simulink subsystem "railCarBrakeSubSystem"  (R2025a)
settings: Solver=VariableStepAuto  StartTime=0.0  StopTime=10.0  RelTol=1e-3
model mask{reservoir_temperature=70, reservoir_temperature_unit=degF, p_init=air_pressure, p_init_unit=psi, r_volume=10, r_volume_unit=gal, bc_volume=4, bc_volume_unit=gal, bc_pressure=14.69, bc_pressure_unit=psi, length=50, length_unit=ft, area=1.23, area_unit=in^2, Dh=1.25, Dh_unit=in}
  mask prompts: reservoir_temperature "physmod:simscape:library:comments:gas:elements:reservoir:reservoir_temperature"; p_init "physmod:simscape:library:comments:gas:elements:pipe:p_init"; r_volume "Volume"; bc_volume "Volume"; bc_pressure "Pressure"; length "Pipe length"; area "Cross-sectional area"; Dh "Hydraulic diameter"
libraries: fl_lib x17, nesl_utility x10, SimscapeFluids_lib x5
settings Model: Creator=adam  LastModifiedBy=adam
settings OptimizationCC: ReuseModelBlockBuffer=off
settings RTWCC: GPUComputeCapability=3.5

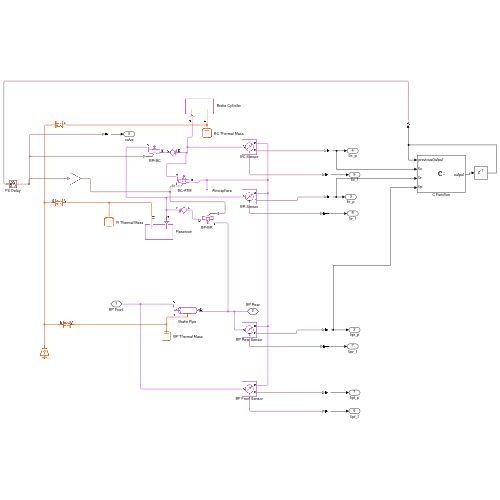
[thumbnail: Simulink's stored preview of the top-level diagram]
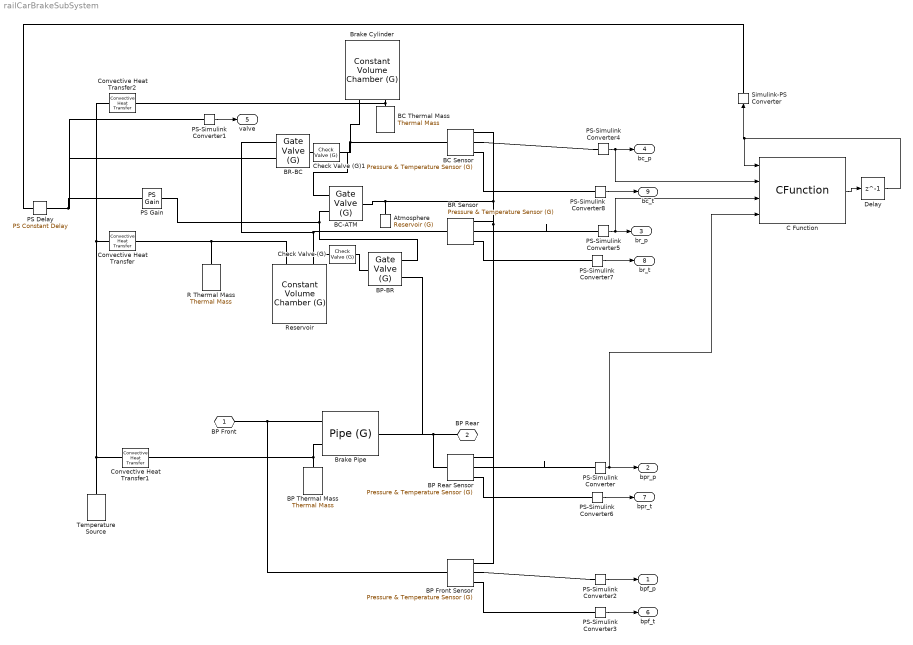
== system railCarBrakeSubSystem ==
  Atmosphere : fl_lib/Gas/Elements/Reservoir (G)  pressure_spec=foundation.enum.pressure_spec.atmospheric  reservoir_pressure=0.101325 MPa  reservoir_temperature=reservoir_temperature degF  area_A=10 ft^2
  BC Sensor : fl_lib/Gas/Sensors/Pressure & Temperature Sensor (G)  reference=foundation.enum.MeasurementReference.difference  pressure=true  pressure_spec=foundation.enum.PressureMeasementSpec.Absolute  temperature=true
      settings: InternalSimscapePortConfiguration="{\"Bottom\":[{\"id\":\"T\",\"label\":\"T\",\"type\":\"output\"}],\"Left\":[{\"id\":\"A\",\"label\":\"A\",\"type\":\"foundation.gas.gas\"}],\"Right\":[{\"id\":\"B\",\"label\":\"B\",\"type\":\"foundation.gas.gas\"},{\"id\":\"P\",\"label\":\"P\",\"type\":\"output\"}],\"Top\":[]}"
  BC Thermal Mass : fl_lib/Thermal/Thermal Elements/Thermal Mass  mass_type=foundation.enum.constant_variable.constant  mass=100 kg  sp_heat=447 J/(K*kg)  mass_min=1e-6 kg  num_ports=foundation.enum.numPorts2.one  m_specify=off  m_priority=High  m=1 kg  m_nominal_specify=off  m_nominal_value=1  m_nominal_unit=kg  T_specify=on  T_priority=High  T=reservoir_temperature degF  T_nominal_specify=off  T_nominal_value=1  T_nominal_unit=K  Q_specify=off  Q_priority=None  Q=0 W  Q_nominal_specify=off  Q_nominal_value=1  Q_nominal_unit=W
  BC-ATM : SimscapeFluids_lib/Gas/Valves & Orifices/Flow Control Valves/Gate Valve (G)  diam_orifice=1.25 in  valve_parameterization=fluids.gas.valves_orifices.flow_control_valves.enum.OrificeParameterization.Cv  Cd=0.64  Cv_max=4  xT_Cv=0.7  Kv_max=3.6  xT_Kv=0.7  C_max=12 l/(bar*s)  B_crit_linear=0.3  m=0.5  T_ref_C=293.15 K  rho_ref_C=1.185 kg/m^3  leakage_fraction=1e-7  smoothing_factor=0.0001  B_lam=0.999  area=1.23 in^2  x0=0
      settings: InternalSimscapePortConfiguration="{\"Bottom\":[],\"Left\":[{\"id\":\"A\",\"label\":\"A\",\"type\":\"foundation.gas.gas\"},{\"id\":\"L\",\"label\":\"L\",\"type\":\"input\"}],\"Right\":[{\"id\":\"B\",\"label\":\"B\",\"type\":\"foundation.gas.gas\"}],\"Top\":[]}"
  BP Front Sensor : fl_lib/Gas/Sensors/Pressure & Temperature Sensor (G)  reference=foundation.enum.MeasurementReference.difference  pressure=true  pressure_spec=foundation.enum.PressureMeasementSpec.Absolute  temperature=true
      settings: InternalSimscapePortConfiguration="{\"Bottom\":[{\"id\":\"T\",\"label\":\"T\",\"type\":\"output\"}],\"Left\":[{\"id\":\"A\",\"label\":\"A\",\"type\":\"foundation.gas.gas\"}],\"Right\":[{\"id\":\"B\",\"label\":\"B\",\"type\":\"foundation.gas.gas\"},{\"id\":\"P\",\"label\":\"P\",\"type\":\"output\"}],\"Top\":[]}"
  BP Rear Sensor : fl_lib/Gas/Sensors/Pressure & Temperature Sensor (G)  reference=foundation.enum.MeasurementReference.difference  pressure=true  pressure_spec=foundation.enum.PressureMeasementSpec.Absolute  temperature=true
      settings: InternalSimscapePortConfiguration="{\"Bottom\":[{\"id\":\"T\",\"label\":\"T\",\"type\":\"output\"}],\"Left\":[{\"id\":\"A\",\"label\":\"A\",\"type\":\"foundation.gas.gas\"}],\"Right\":[{\"id\":\"B\",\"label\":\"B\",\"type\":\"foundation.gas.gas\"},{\"id\":\"P\",\"label\":\"P\",\"type\":\"output\"}],\"Top\":[]}"
  BP Thermal Mass : fl_lib/Thermal/Thermal Elements/Thermal Mass  mass_type=foundation.enum.constant_variable.constant  mass=2.27*50 lbm  sp_heat=447 J/(K*kg)  mass_min=1e-6 kg  num_ports=foundation.enum.numPorts2.one  m_specify=off  m_priority=High  m=1 kg  m_nominal_specify=off  m_nominal_value=1  m_nominal_unit=kg  T_specify=on  T_priority=High  T=reservoir_temperature degF  T_nominal_specify=off  T_nominal_value=1  T_nominal_unit=K  Q_specify=off  Q_priority=None  Q=0 W  Q_nominal_specify=off  Q_nominal_value=1  Q_nominal_unit=W
  BP-BR : SimscapeFluids_lib/Gas/Valves & Orifices/Flow Control Valves/Gate Valve (G)  diam_orifice=1.25 in  valve_parameterization=fluids.gas.valves_orifices.flow_control_valves.enum.OrificeParameterization.Cv  Cd=0.64  Cv_max=4  xT_Cv=0.7  Kv_max=3.6  xT_Kv=0.7  C_max=12 l/(bar*s)  B_crit_linear=0.3  m=0.5  T_ref_C=293.15 K  rho_ref_C=1.185 kg/m^3  leakage_fraction=1e-7  smoothing_factor=0.0001  B_lam=0.999  area=1.23 in^2  x0=0
      settings: InternalSimscapePortConfiguration="{\"Bottom\":[],\"Left\":[{\"id\":\"A\",\"label\":\"A\",\"type\":\"foundation.gas.gas\"},{\"id\":\"L\",\"label\":\"L\",\"type\":\"input\"}],\"Right\":[{\"id\":\"B\",\"label\":\"B\",\"type\":\"foundation.gas.gas\"}],\"Top\":[]}"
  BR Sensor : fl_lib/Gas/Sensors/Pressure & Temperature Sensor (G)  reference=foundation.enum.MeasurementReference.difference  pressure=true  pressure_spec=foundation.enum.PressureMeasementSpec.Absolute  temperature=true
      settings: InternalSimscapePortConfiguration="{\"Bottom\":[{\"id\":\"T\",\"label\":\"T\",\"type\":\"output\"}],\"Left\":[{\"id\":\"A\",\"label\":\"A\",\"type\":\"foundation.gas.gas\"}],\"Right\":[{\"id\":\"B\",\"label\":\"B\",\"type\":\"foundation.gas.gas\"},{\"id\":\"P\",\"label\":\"P\",\"type\":\"output\"}],\"Top\":[]}"
  BR-BC : SimscapeFluids_lib/Gas/Valves & Orifices/Flow Control Valves/Gate Valve (G)  diam_orifice=1.25 in  valve_parameterization=fluids.gas.valves_orifices.flow_control_valves.enum.OrificeParameterization.Cv  Cd=0.64  Cv_max=4  xT_Cv=0.7  Kv_max=3.6  xT_Kv=0.7  C_max=12 l/(bar*s)  B_crit_linear=0.3  m=0.5  T_ref_C=293.15 K  rho_ref_C=1.185 kg/m^3  leakage_fraction=1e-7  smoothing_factor=0.0001  B_lam=0.999  area=1.23 in^2  x0=0
      settings: InternalSimscapePortConfiguration="{\"Bottom\":[],\"Left\":[{\"id\":\"A\",\"label\":\"A\",\"type\":\"foundation.gas.gas\"},{\"id\":\"L\",\"label\":\"L\",\"type\":\"input\"}],\"Right\":[{\"id\":\"B\",\"label\":\"B\",\"type\":\"foundation.gas.gas\"}],\"Top\":[]}"
  Brake Cylinder : fl_lib/Gas/Elements/Constant Volume Chamber (G)  volume=bc_volume gal  num_ports=foundation.enum.num_ports.one  area_A=0.11 in^2  area_B=0.11 in^2  area_C=0.01 m^2  area_D=0.01 m^2  p_I_specify=on  p_I_priority=High  p_I=bc_pressure psi  p_I_nominal_specify=off  p_I_nominal_value=1  p_I_nominal_unit=MPa  T_I_specify=on  T_I_priority=High  T_I=reservoir_temperature degF  T_I_nominal_specify=off  T_I_nominal_value=1  T_I_nominal_unit=K  rho_I_specify=off  rho_I_priority=None  rho_I=1.2 kg/m^3  rho_I_nominal_specify=off  rho_I_nominal_value=1  rho_I_nominal_unit=kg/m^3
      settings: InternalSimscapePortConfiguration="{\"Bottom\":[],\"Left\":[{\"id\":\"A\",\"label\":\"A\",\"type\":\"foundation.gas.gas\"},{\"id\":\"H\",\"label\":\"H\",\"type\":\"foundation.thermal.thermal\"}],\"Right\":[],\"Top\":[]}"
  Brake Pipe : fl_lib/Gas/Elements/Pipe (G)  length=length ft  area=area in^2  Dh=Dh in  length_add=0.1 m  roughness=15e-6 m  Re_lam=2000  Re_tur=4000  shape_factor=64  Nu_lam=3.66  dynamic_compressibility=true  inertia=false  p_init=p_init psi  p_init_priority=foundation.enum.Priority.High  T_init=reservoir_temperature degF  T_init_priority=foundation.enum.Priority.High  mdot_init=0 kg/s  mdot_init_priority=foundation.enum.Priority.High  p_nominal=0.101325 MPa  T_nominal=293.15 K
  C Function : CFunction  OutputCode=|  GenerateCodeAsIs=off  CodegenOutputCode=|  CustomCodeSettingLocation=ModelConfigurationParameters
      OutputCode=|
      | // 1 = Apply
      | // 0 = Lap
      | // -1 = Release
      | 
      | if (bp > br + 1.5) {
      |     // BP-BR and BC-ATM
      |     output = -1;
      | } else if (bp < br - 1.5) {
      |     // BR-BC
      |     output = 1;
      | } else {
      |     output = 0;   
      | }
      CodegenOutputCode=|
      | // 1 = Apply
      | // 0 = Lap
      | // -1 = Release
      | 
      | if (bp > br + 1.5) {
      |     // BP-BR and BC-ATM
      |     output = -1;
      | } else if (bp < br - 1.5) {
      |     // BR-BC
      |     output = 1;
      | } else {
      |     output = 0;   
      | }
  Check Valve (G) : SimscapeFluids_lib/Gas/Valves & Orifices/Directional Control Valves/Check Valve (G)  opening_pressure_spec=fluids.gas.valves_orifices.enum.PressureControlSpec.PressureDifference  p_crack_differential=0.1 psi  p_crack_gauge=0.1 MPa  press_max_differential=0.25 psi  press_max_gauge=0.2 MPa  valve_parameterization=fluids.gas.valves_orifices.enum.OrificeParameterization.Cv  Cv_max=4  xT_Cv=0.7  Kv_max=3.6  xT_Kv=0.7  C_max=12 l/(bar*s)  B_crit_linear=0.3  m=0.5  T_ref_C=293.15 K  rho_ref_C=1.185 kg/m^3  orifice_area_max=1e-4 m^2  Cd=0.64  leakage_fraction=1e-7  smoothing_factor=0.01  B_lam=0.999  area=1.23 in^2
      settings: InternalSimscapePortConfiguration="{\"Bottom\":[],\"Left\":[{\"id\":\"A\",\"label\":\"A\",\"type\":\"foundation.gas.gas\"}],\"Right\":[{\"id\":\"B\",\"label\":\"B\",\"type\":\"foundation.gas.gas\"}],\"Top\":[]}"
  Check Valve (G)1 : SimscapeFluids_lib/Gas/Valves & Orifices/Directional Control Valves/Check Valve (G)  opening_pressure_spec=fluids.gas.valves_orifices.enum.PressureControlSpec.PressureDifference  p_crack_differential=0.1 psi  p_crack_gauge=0.1 MPa  press_max_differential=0.25 psi  press_max_gauge=0.2 MPa  valve_parameterization=fluids.gas.valves_orifices.enum.OrificeParameterization.Cv  Cv_max=4  xT_Cv=0.7  Kv_max=3.6  xT_Kv=0.7  C_max=12 l/(bar*s)  B_crit_linear=0.3  m=0.5  T_ref_C=293.15 K  rho_ref_C=1.185 kg/m^3  orifice_area_max=1e-4 m^2  Cd=0.64  leakage_fraction=1e-7  smoothing_factor=0.01  B_lam=0.999  area=1.23 in^2
      settings: InternalSimscapePortConfiguration="{\"Bottom\":[],\"Left\":[{\"id\":\"A\",\"label\":\"A\",\"type\":\"foundation.gas.gas\"}],\"Right\":[{\"id\":\"B\",\"label\":\"B\",\"type\":\"foundation.gas.gas\"}],\"Top\":[]}"
  Convective Heat Transfer : fl_lib/Thermal/Thermal Elements/Convective Heat Transfer  thermal_type=foundation.enum.constant_variable.constant  area=2*pi*0.66*1.25+2*pi*(0.66^2) ft^2  heat_tr_coeff=20 W/(K*m^2)  min_heat_tr_coeff=1e-3 W/(K*m^2)  T_specify=off  T_priority=None  T=0 K  T_nominal_specify=off  T_nominal_value=1  T_nominal_unit=K  Q_specify=off  Q_priority=None  Q=0 W  Q_nominal_specify=off  Q_nominal_value=1  Q_nominal_unit=W
  Convective Heat Transfer1 : fl_lib/Thermal/Thermal Elements/Convective Heat Transfer  thermal_type=foundation.enum.constant_variable.constant  area=2*sqrt(pi*area) * length ft^2  heat_tr_coeff=20 W/(K*m^2)  min_heat_tr_coeff=1e-3 W/(K*m^2)  T_specify=off  T_priority=None  T=0 K  T_nominal_specify=off  T_nominal_value=1  T_nominal_unit=K  Q_specify=off  Q_priority=None  Q=0 W  Q_nominal_specify=off  Q_nominal_value=1  Q_nominal_unit=W
  Convective Heat Transfer2 : fl_lib/Thermal/Thermal Elements/Convective Heat Transfer  thermal_type=foundation.enum.constant_variable.constant  area=2*pi*0.66*1.25+2*pi*(0.66^2) ft^2  heat_tr_coeff=20 W/(K*m^2)  min_heat_tr_coeff=1e-3 W/(K*m^2)  T_specify=off  T_priority=None  T=0 K  T_nominal_specify=off  T_nominal_value=1  T_nominal_unit=K  Q_specify=off  Q_priority=None  Q=0 W  Q_nominal_specify=off  Q_nominal_value=1  Q_nominal_unit=W
  Delay : Delay  DelayLength=1  InitialCondition=0
  PS Delay : fl_lib/Physical Signals/Delays/PS Constant Delay  InputHistory=0.0  DelayTime=0.001 s
      settings: InternalSimscapePortConfiguration="{\"Bottom\":[],\"Left\":[{\"id\":\"U\",\"label\":\"U\",\"type\":\"input\"}],\"Right\":[{\"id\":\"Y\",\"label\":\"Y\",\"type\":\"output\"}],\"Top\":[]}"
  PS Gain : fl_lib/Physical Signals/Functions/PS Gain  gain=-1
  PS-Simulink Converter{,2,4..5} (4 alike) : nesl_utility/PS-Simulink Converter  PhysicalDomain=network_engine_domain  SubClassName=ps_output  LeftPortType=input  RightPortType=output  PseudoPeriodic=off  Frequencies=[]  VectorFormat=inherit  Unit=psi  AffineConversion=off
  PS-Simulink Converter1 : nesl_utility/PS-Simulink Converter  PhysicalDomain=network_engine_domain  SubClassName=ps_output  LeftPortType=input  RightPortType=output  PseudoPeriodic=off  Frequencies=[]  VectorFormat=inherit  Unit=inherit  AffineConversion=off
  PS-Simulink Converter{3,6..8} (4 alike) : nesl_utility/PS-Simulink Converter  PhysicalDomain=network_engine_domain  SubClassName=ps_output  LeftPortType=input  RightPortType=output  PseudoPeriodic=off  Frequencies=[]  VectorFormat=inherit  Unit=degC  AffineConversion=on
  R Thermal Mass : fl_lib/Thermal/Thermal Elements/Thermal Mass  mass_type=foundation.enum.constant_variable.constant  mass=100 kg  sp_heat=447 J/(K*kg)  mass_min=1e-6 kg  num_ports=foundation.enum.numPorts2.one  m_specify=off  m_priority=High  m=1 kg  m_nominal_specify=off  m_nominal_value=1  m_nominal_unit=kg  T_specify=on  T_priority=High  T=reservoir_temperature degF  T_nominal_specify=off  T_nominal_value=1  T_nominal_unit=K  Q_specify=off  Q_priority=None  Q=0 W  Q_nominal_specify=off  Q_nominal_value=1  Q_nominal_unit=W
  Reservoir : fl_lib/Gas/Elements/Constant Volume Chamber (G)  volume=r_volume gal  num_ports=foundation.enum.num_ports.one  area_A=0.12 in^2  area_B=0.11 in^2  area_C=0.01 m^2  area_D=0.01 m^2  p_I_specify=on  p_I_priority=High  p_I=p_init psi  p_I_nominal_specify=off  p_I_nominal_value=1  p_I_nominal_unit=MPa  T_I_specify=on  T_I_priority=High  T_I=reservoir_temperature degF  T_I_nominal_specify=off  T_I_nominal_value=1  T_I_nominal_unit=K  rho_I_specify=off  rho_I_priority=None  rho_I=1.2 kg/m^3  rho_I_nominal_specify=off  rho_I_nominal_value=1  rho_I_nominal_unit=kg/m^3
      settings: InternalSimscapePortConfiguration="{\"Bottom\":[],\"Left\":[{\"id\":\"A\",\"label\":\"A\",\"type\":\"foundation.gas.gas\"},{\"id\":\"H\",\"label\":\"H\",\"type\":\"foundation.thermal.thermal\"}],\"Right\":[],\"Top\":[]}"
  Simulink-PS Converter : nesl_utility/Simulink-PS Converter  PhysicalDomain=network_engine_domain  SubClassName=ps_input  LeftPortType=input  RightPortType=output  PseudoPeriodic=off  Frequencies=[]  NoiseDistribution=none  NoiseParameters=[]  Unit=1  AffineConversion=off  FilteringAndDerivatives=provide  SimscapeFilterOrder=1  InputFilterTimeConstant=0.001  UdotUserProvided=0
  Temperature Source : fl_lib/Thermal/Thermal Sources/Temperature Source  temperature=reservoir_temperature degF
  BP Front : PMIOPort  Side=Left
  BP Rear : PMIOPort  Port=2  Side=Left
  bpf_p : Outport
  bpr_p : Outport  Port=2
  br_p : Outport  Port=3
  bc_p : Outport  Port=4
  valve : Outport  Port=5
  bpf_t : Outport  Port=6
  bpr_t : Outport  Port=7
  br_t : Outport  Port=8
  bc_t : Outport  Port=9
  wires:
  PS-Simulink Converter/1 -> C Function/4, bpr_p/1
  PS-Simulink Converter2/1 -> bpf_p/1
  PS-Simulink Converter4/1 -> bc_p/1, C Function/2
  C Function/1 -> Delay/1
  Delay/1 -> C Function/1, Simulink-PS Converter/1
  PS-Simulink Converter5/1 -> br_p/1, C Function/3
  PS-Simulink Converter1/1 -> valve/1
  PS-Simulink Converter3/1 -> bpf_t/1
  PS-Simulink Converter6/1 -> bpr_t/1
  PS-Simulink Converter7/1 -> br_t/1
  PS-Simulink Converter8/1 -> bc_t/1
  connections:
  Convective Heat Transfer/LConn1 -- R Thermal Mass/LConn1 -- Reservoir/LConn2
  BP Front/RConn1 -- BP Front Sensor/LConn1 -- Brake Pipe/LConn1
  Atmosphere/LConn1 -- BC Sensor/RConn1 -- BR Sensor/RConn1 -- BP Rear Sensor/RConn1 -- BP Front Sensor/RConn1 -- BC-ATM/RConn1
  BP Thermal Mass/LConn1 -- Brake Pipe/LConn2 -- Convective Heat Transfer1/LConn1
  Brake Cylinder/LConn2 -- Convective Heat Transfer2/LConn1 -- BC Thermal Mass/LConn1
  BP Rear Sensor/LConn1 -- Brake Pipe/RConn1 -- BP-BR/LConn1 -- BP Rear/RConn1
  Convective Heat Transfer/RConn1 -- Convective Heat Transfer1/RConn1 -- Temperature Source/LConn1 -- Convective Heat Transfer2/RConn1
  BR Sensor/LConn1 -- Check Valve (G)/RConn1 -- Reservoir/LConn1 -- BR-BC/LConn1
  Brake Cylinder/LConn1 -- Check Valve (G)1/RConn1 -- BC-ATM/LConn1 -- BC Sensor/LConn1
  BP Rear Sensor/RConn2 -- PS-Simulink Converter/LConn1
  BC Sensor/RConn2 -- PS-Simulink Converter4/LConn1
  BP Front Sensor/RConn2 -- PS-Simulink Converter2/LConn1
  BP-BR/LConn2 -- PS Gain/RConn1 -- BC-ATM/LConn2
  PS Delay/LConn1 -- Simulink-PS Converter/RConn1
  BR Sensor/RConn2 -- PS-Simulink Converter5/LConn1
  BP-BR/RConn1 -- Check Valve (G)/LConn1
  BR-BC/RConn1 -- Check Valve (G)1/LConn1
  BR-BC/LConn2 -- PS-Simulink Converter1/LConn1 -- PS Gain/LConn1 -- PS Delay/RConn1
  BP Front Sensor/RConn3 -- PS-Simulink Converter3/LConn1
  BP Rear Sensor/RConn3 -- PS-Simulink Converter6/LConn1
  BR Sensor/RConn3 -- PS-Simulink Converter7/LConn1
  BC Sensor/RConn3 -- PS-Simulink Converter8/LConn1
